simulink model "simulacaoPPP"  (R2016a)
settings: Solver=VariableStepAuto  StartTime=0.0  StopTime=20  RelTol=1e-3
values from neighbouring files (symbols this model uses):
  m3 = 3.12    [PPP_controle.m]
  m4 = 0.2    [PPP_controle.m]
  Ponto1 = [5 5 -16 1]    [PPP_controle.m]
undefined symbols (not defined in the file or in its folder): D1, D2, N1, N2
settings Model: Creator=bruna  LastModifiedBy=bruna

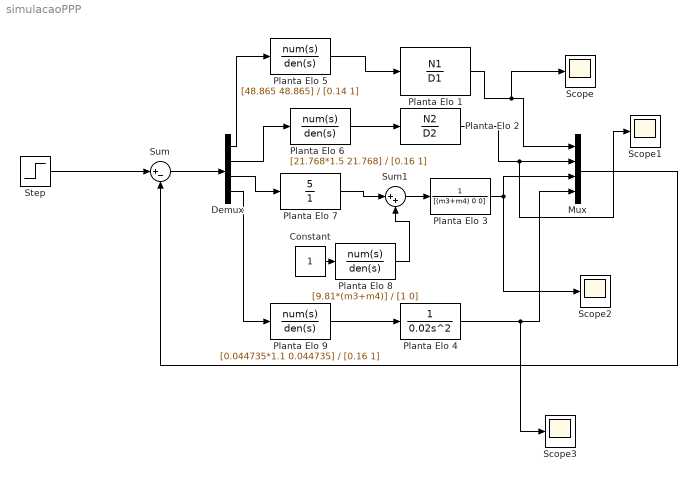
== system simulacaoPPP ==
  Constant : Constant
  Demux : Demux
  Mux : Mux
  Planta Elo 1 : TransferFcn  Numerator=N1  Denominator=D1
  Planta Elo 2 : TransferFcn  Numerator=N2  Denominator=D2
  Planta Elo 3 : TransferFcn  Denominator=[(m3+m4) 0 0]
  Planta Elo 4 : TransferFcn  Denominator=[0.02 0 0]
  Planta Elo 5 : TransferFcn  Numerator=[48.865 48.865]  Denominator=[0.14 1]
  Planta Elo 6 : TransferFcn  Numerator=[21.768*1.5 21.768]  Denominator=[0.16 1]
  Planta Elo 7 : TransferFcn  Numerator=[5]  Denominator=[1]
  Planta Elo 8 : TransferFcn  Numerator=[9.81*(m3+m4)]  Denominator=[1 0]
  Planta Elo 9 : TransferFcn  Numerator=[0.044735*1.1 0.044735]  Denominator=[0.16 1]
  Scope{,1..3} (4 alike) : Scope
  Step : Step  After=Ponto1  SampleTime=0
  Sum : Sum  Inputs=|+-
  Sum1 : Sum  Inputs=|++
  wires:
  Sum/1 -> Demux/1
  Demux/1 -> Planta Elo 5/1
  Demux/3 -> Planta Elo 7/1
  Demux/4 -> Planta Elo 9/1
  Planta Elo 5/1 -> Planta Elo 1/1
  Planta Elo 9/1 -> Planta Elo 4/1
  Planta Elo 2/1 -> Scope1/1, Mux/2
  Planta Elo 3/1 -> Mux/3, Scope2/1
  Planta Elo 4/1 -> Scope3/1, Mux/4
  Mux/1 -> Sum/2
  Planta Elo 1/1 -> Scope/1, Mux/1
  Step/1 -> Sum/1
  Planta Elo 6/1 -> Planta Elo 2/1
  Demux/2 -> Planta Elo 6/1
  Sum1/1 -> Planta Elo 3/1
  Planta Elo 7/1 -> Sum1/1
  Constant/1 -> Planta Elo 8/1
  Planta Elo 8/1 -> Sum1/2
